simulink model "Proyecto"  (R2023b)
settings: Solver=VariableStepAuto  StartTime=0.0  StopTime=29  FixedStep=1/100000  RelTol=1e-3
libraries: simulink x3, robotmobilelib x1
settings Model: SimulationMode=accelerator  Creator=rubencruzgonzalez  LastModifiedBy=rubencruzgonzalez
settings OptimizationCC: DefaultParameterBehavior=Inlined  EnhancedBackFolding=on  PassReuseOutputArgsAs=Individual arguments  ZeroExternalMemoryAtStartup=off  ZeroInternalMemoryAtStartup=off  OptimizeBlockOrder=speed  DifferentSizesBufferReuse=on  OptimizationCustomize=off  EfficientTunableParamExpr=on
settings DebuggingCC: ParameterTunabilityLossMsg=error
settings HardwareCC: ProdBitPerLong=64  ProdHWDeviceType=Intel->x86-64 (Mac OS X)
settings SFSimCC: MATLABDynamicMemAlloc=off
settings RTWCC: Description=Embedded Coder  SystemTargetFile=ert.tlc  TemplateMakefile=ert_default_tmf
settings CodeAppCC: ForceParamTrailComments=on  IgnoreCustomStorageClasses=off  OperatorAnnotations=on  SimulinkDataObjDesc=on  SFDataObjDesc=on  InsertBlockDesc=on
settings ERTTargetCC: TargetLangStandard=C99 (ISO)  GenerateSampleERTMain=on  InlinedParameterPlacement=NonHierarchical  ERTCustomFileTemplate=example_file_process.tlc

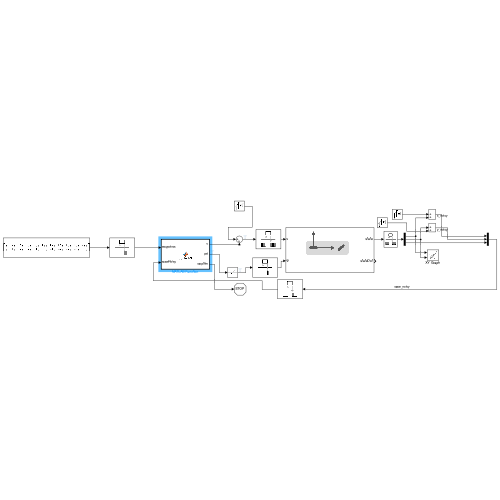
[thumbnail: Simulink's stored preview of the top-level diagram]
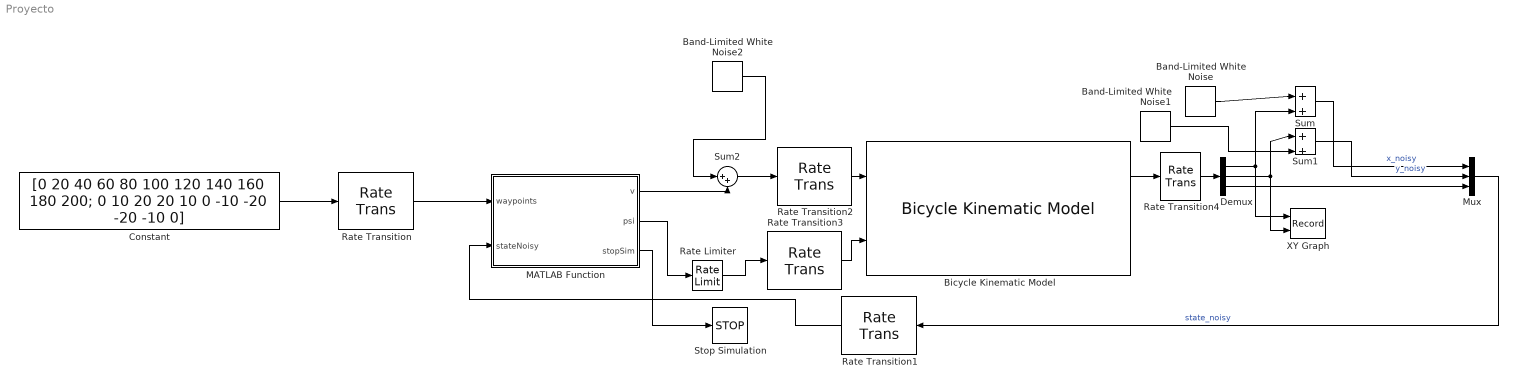
== system Proyecto ==
  Band-Limited White Noise : simulink/Sources/Band-Limited White Noise  Tag=noise_x  Cov=[0.01]  Ts=1/100  seed=[23341]
  Band-Limited White Noise1 : simulink/Sources/Band-Limited White Noise  Tag=noise_y  Cov=[0.01]  Ts=1/100  seed=[23341]
  Band-Limited White Noise2 : simulink/Sources/Band-Limited White Noise  Tag=noise_x  Cov=[0.001]  Ts=1/100000  seed=[23341]
  Bicycle Kinematic Model : robotmobilelib/Bicycle Kinematic Model  VehicleInputs=Vehicle Speed & Steering Angle  WheelBase=1  VehicleSpeedRange=[0 30]  MaxSteeringAngle=pi/4  InitialState=[0; 0; 0]  SimulateUsing=Code generation
  Constant : Constant  Value=|
      | [0    20   40   60   80   100  120  140  160  180  200;
      |  0    10   20   20   10    0   -10  -20  -20  -10    0]
  Demux : Demux  Outputs=3
  MATLAB Function : MATLAB Function  TreatAsAtomicUnit=on
  Mux : Mux  Inputs=3
  Rate Limiter : RateLimiter  RisingSlewLimit=pi/4  FallingSlewLimit=-pi/4  SampleTimeMode=inherited
  Rate Transition : RateTransition  OutPortSampleTime=1/100
  Rate Transition1 : RateTransition  OutPortSampleTime=1/100
  Rate Transition2 : RateTransition  OutPortSampleTime=1/1000
  Rate Transition3 : RateTransition  OutPortSampleTime=1/1000
  Rate Transition4 : RateTransition  OutPortSampleTime=1/1000
  Stop Simulation : Stop
  Sum : Sum  Inputs=|++
  Sum1 : Sum  Inputs=|++
  Sum2 : Sum  Inputs=|++
  XY Graph : Record  FileSettingsInternal="{\"entries\":[{\"content\":{\"excelSettings\":{\"content\":{},\"type\":\"Streamout.ExcelSettings\"}},\"type\":\"Streamout.FileSettingStorage\",\"uuid\":\"\"}],\"packageUris\":[\"http:\\/\\/schema.mathworks.com\\/mf0\\/streamout_blocks\\/R2020a\"],\"version\":\"1.0\"}"  Layout=[1 1]  SignalsInternal="{\"entries\":[{\"content\":{\"signals\":[{\"content\":{\"blockPath\":[],\"dimensions\":[1],\"domain\":\"\",\"lineColor\":\"#a2142f\",\"plots\":[1],\"port\":1,\"signalID\":16,\"signalName\":\"Demux:1\"},\"type\":\"RecordBlkView.Signal\",\"uuid\":\"\"},{\"content\":{\"blockPath\":[],\"dimensions\":[1],\"domain\":\"\",\"lineColor\":\"#139fff\",\"plots\":[1],\"port\":2,\"signalID\":19,\"signalName\":\"Demux:2\"},\"type\":\"RecordBlkView.Signal\",\"uuid\":\"\"}]},\"type\":\"RecordBlkView.InputSignals\",\"uuid\":\"\"}],\"packageUris\":[\"http:\\/\\/schema.mathworks.com\\/mf0\\/streamout_blocks\\/R2020a\"],\"version\":\"1.0\"}"  VisualizationBindings="{\"xyplotplugin\":{\"info\":[{\"series\":[{\"bindingParametersList\":[{\"parameter\":\"X-Axis\",\"signalID\":16,\"signalName\":\"Demux:1\"},{\"parameter\":\"Y-Axis\",\"signalID\":19,\"signalName\":\"Demux:2\"}],\"seriesID\":60465}],\"subplotID\":1}]}}"  CompatibilityTag=XY
  wires:
  MATLAB Function/2(psi) -> Rate Limiter/1
  Bicycle Kinematic Model/1 -> Rate Transition4/1
  Demux/1 -> XY Graph/1, Sum/2
  Band-Limited White Noise/1 -> Sum/1
  Band-Limited White Noise1/1 -> Sum1/2
  Demux/2 -> XY Graph/2, Sum1/1
  Demux/3 -> Mux/3
  Mux/1 -> Rate Transition1/1  "state_noisy"
  Sum1/1 -> Mux/2  "y_noisy"
  Sum/1 -> Mux/1  "x_noisy"
  MATLAB Function/3(stopSim) -> Stop Simulation/1
  Constant/1 -> Rate Transition/1
  Rate Transition/1 -> MATLAB Function/1(waypoints)
  Rate Transition1/1 -> MATLAB Function/2(stateNoisy)
  Rate Transition2/1 -> Bicycle Kinematic Model/1
  Rate Transition3/1 -> Bicycle Kinematic Model/2
  Rate Transition4/1 -> Demux/1
  Rate Limiter/1 -> Rate Transition3/1
  Sum2/1 -> Rate Transition2/1
  Band-Limited White Noise2/1 -> Sum2/1
  MATLAB Function/1(v) -> Sum2/2

== matlab function Proyecto/MATLAB Function ==
  settings: updateMethod=DISCRETE
  data: v output; waypoints input; psi output; stateNoisy input; stopSim output
function [v, psi, stopSim] = controlPI(waypoints, stateNoisy)
    % CONTROLPI: Controlador PI de la orientación + índice persistente
    % para avanzar entre varios waypoints.
    %
    % Entradas:
    %   - waypoints: matriz 2xN con las coordenadas [x; y] de los puntos.
    %   - stateNoisy: vector [x_noisy, y_noisy, theta] con ruido.
    %
    % Salidas:
    %   - v: velocidad del vehículo
    %   - psi: ángulo de dirección
    %   - stopSim: señal booleana (1 para detener simulación)

    % ========== 1) ÍNDICE PERSISTENTE PARA WAYPOINTS ==========
    persistent idx;
    if isempty(idx)
        idx = 1;  % Iniciamos en el primer waypoint
    end

    % ========== 2) VARIABLES PERSISTENTES PARA EL CONTROL INTEGRAL ==========
    persistent error_orient_integral;
    if isempty(error_orient_integral)
        error_orient_integral = 0;  % Acumulador de error
    end

    % ========== 3) PARÁMETROS ==========
    % Ganancias PI
    Kp = 2;    % Ganancia proporcional
    Ki = 0.001;    % Ganancia integral (ajusta según necesites)
    % Threshold para detectar llegada a un waypoint
    threshold = 0.5;
    % Velocidad fija
    v = 10;
    % Por defecto, no paramos la simulación
    stopSim = 0;

    % ========== 4) OBTENER POSICIÓN Y ORIENTACIÓN ACTUAL ==========
    x_actual = stateNoisy(1);
    y_actual = stateNoisy(2);
    theta_actual = stateNoisy(3);

    % ========== 5) VERIFICAR SI YA PASAMOS EL ÚLTIMO WAYPOINT ==========
    if idx > size(waypoints, 2)
        % Si ya no hay más waypoints, paramos el vehículo
        v = 0;
        psi = 0;
        % Opcional: señal para detener simulación
        stopSim = 1;
        return;
    end

    % ========== 6) WAYPOINT ACTUAL ==========
    x_ref = waypoints(1, idx);
    y_ref = waypoints(2, idx);

    % ========== 7) CÁLCULO DE DISTANCIA AL WAYPOINT ACTUAL ==========
    error_x = x_ref - x_actual;
    error_y = y_ref - y_actual;
    dist = sqrt(error_x^2 + error_y^2);

    % Cuando estamos lo bastante cerca, avanzamos al siguiente waypoint
    if dist < threshold && idx < size(waypoints, 2)
        idx = idx + 1;
    end

    % ========== 8) CÁLCULO DE ERROR DE ORIENTACIÓN ==========
    angulo_deseado = atan2(error_y, error_x);
    error_orientacion = angulo_deseado - theta_actual;
    % Ajustar error en el rango [-pi, pi]
    error_orientacion = atan2(sin(error_orientacion), cos(error_orientacion));

    % ========== 9) ACUMULACIÓN DEL ERROR (PARTE INTEGRAL) ==========
    % Aquí se asume un paso de simulación pequeño. Para ser más riguroso,
    % podrías multiplicar por Ts (el paso de tiempo), si lo conoces.

    Ts = 1/100;
    error_orient_integral = error_orient_integral + (error_orientacion*Ts);
    

    % ========== 10) LEY DE CONTROL PI ==========
    psi_control = Kp * error_orientacion + Ki * error_orient_integral;

    % ========== 11) SATURACIÓN DEL ÁNGULO DE DIRECCIÓN ==========
    % Limitar entre ±45° (±pi/4)
    psi = max(min(psi_control, pi/16), -pi/16);
end
